simulink model "allstates_chart"  (R2015b)
settings: Solver=VariableStepAuto  StartTime=0.0  StopTime=10.0  RelTol=1e-3
settings Model: Creator=Gabriel  LastModifiedBy=Gabriel

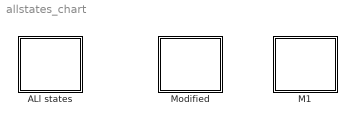
== system allstates_chart ==
  ALl states : Stateflow chart  TreatAsAtomicUnit=on
  "M1 " : Stateflow chart  TreatAsAtomicUnit=on
  Modified : Stateflow chart  TreatAsAtomicUnit=on

== stateflow chart allstates_chart/Modified ==
  state IEI
  note: I = Idle
      | E = Empty
      | P = Processing
      | F = Full
      | D = Down
  state IED
  state PEI
  state DEI
  state IFI
  state IEP
  state DED
  state IFD
  state PEP
  state IFP
  state PED
  DEI -> IEI
  IEP -> IEI [order 2]
  IED -> IEI
  IEI -> PEI
  PEI -> DEI [order 1]
  PED -> PEI [order 3]
  IEP -> IED [order 1]
  PEI -> IFI [order 2]
  DED -> DEI
  IFD -> IFI
  IFI -> IEP
  IFP -> IEP [order 2]
  IEP -> PEP [order 3]
  PEP -> DED [order 1]
  PED -> DED [order 2]
  PEP -> PED [order 3]
  PED -> IFD [order 1]
  IFP -> IFD [order 1]
  PEP -> IFP [order 2]

== stateflow chart allstates_chart/M1  ==
  note: M1 and M2
  state Processing
  state Idle
  state Down
  note: Buffer
  state Empty
  state Full
  Idle -> Processing : Start
  Processing -> Down [order 1] : Breakdown
  (default) -> Idle [order 1]
  Down -> Idle : Repair
  Processing -> Idle [order 2] : End
  Empty -> Full : Placed
  (default) -> Empty [order 2]
  Full -> Empty : Taken

== stateflow chart allstates_chart/ALl states ==
  state IED
  state IEI
  note: I = Idle
      | E = Empty
      | P = Processing
      | F = Full
      | D = Down
  state IEP
  state PEI
  state DEI
  state IFI
  state PFI
  state DEP
  state IFP
  state DFP
  state PEP
  state PFP
  state DED
  state PED
  state PFD
  state DFD
  state DFI
  state IFD
  DED -> IEI [order 3]
  DED -> IED [order 2]
  DEP -> IEI [order 2]
  DEI -> IEI
  IED -> IEI
  IFP -> IEI [order 1]
  IEP -> IEI [order 1]
  IEP -> IED [order 2]
  IEI -> PEI
  IEP -> PEI [order 3]
  DED -> DEI [order 1]
  PEI -> DEI [order 1]
  PEI -> IFI [order 2]
  IFI -> IEP [order 1]
  PEI -> PFI [order 3]
  PED -> PEI [order 4]
  DEP -> DEI [order 1]
  DFP -> IFI [order 2]
  IFD -> IFI [order 1]
  PFD -> PFI [order 2]
  DFI -> IFI [order 2]
  PFI -> DEP [order 1]
  DFD -> IFI [order 3]
  IFI -> PEP [order 2]
  DEP -> DED [order 3]
  PFI -> PEP [order 2]
  PFI -> PFP [order 3]
  DFI -> DEP [order 1]
  DFP -> DEP [order 1]
  IFP -> DFP [order 2]
  PEP -> IFP [order 3]
  PFP -> DFP [order 2]
  PEP -> DED [order 1]
  PEP -> PED [order 2]
  PFP -> PFD [order 1]
  PED -> DED [order 3]
  PED -> PFD [order 1]
  PED -> IFD [order 2]
  IFD -> PFD [order 2]
  PFD -> DFD [order 1]
  DFD -> DFI [order 2]
  DFD -> IFD [order 1]
